simulink model "AirCtl_Mon"  (R2016b)
settings: configuration reference "CodeGenConfigSet" (kept outside this file)
values from neighbouring files (symbols this model uses):
  AirCtl_dnEngTrans_C = Calibration.Parameter    [init_AirCtl_Mon.m]    (also in init_AirCtl_Mon_SIL.m = Simulink.Parameter)
  AirCtl_dqLeadTrans_C = Calibration.Parameter    [init_AirCtl_Mon.m]    (also in init_AirCtl_Mon_SIL.m = Simulink.Parameter)
  AirCtl_drAPPTrans_C = Calibration.Parameter    [init_AirCtl_Mon.m]    (also in init_AirCtl_Mon_SIL.m = Simulink.Parameter)
  AirCtl_facActDesVal_C = Calibration.Parameter    [init_AirCtl_Mon.m]    (also in init_AirCtl_Mon_SIL.m = Simulink.Parameter)
  AirCtl_facEngTempSmkHysCor_CUR = Calibration.Parameter    [init_AirCtl_Mon.m]    (also in init_AirCtl_Mon_SIL.m = Simulink.Parameter)
  AirCtl_facEngTempSmkHysCor_CURX = Calibration.Parameter    [init_AirCtl_Mon.m]    (also in init_AirCtl_Mon_SIL.m = Simulink.Parameter)
  AirCtl_facEnvPresSmkHysCor_CUR = Calibration.Parameter    [init_AirCtl_Mon.m]    (also in init_AirCtl_Mon_SIL.m = Simulink.Parameter)
  AirCtl_facEnvPresSmkHysCor_CURX = Calibration.Parameter    [init_AirCtl_Mon.m]    (also in init_AirCtl_Mon_SIL.m = Simulink.Parameter)
  AirCtl_mMaxDvt_MAP = Calibration.Parameter    [init_AirCtl_Mon.m]    (also in init_AirCtl_Mon_SIL.m = Simulink.Parameter)
  AirCtl_mMaxDvt_MAPX = Calibration.Parameter    [init_AirCtl_Mon.m]    (also in init_AirCtl_Mon_SIL.m = Simulink.Parameter)
  AirCtl_mMaxDvt_MAPY = Calibration.Parameter    [init_AirCtl_Mon.m]    (also in init_AirCtl_Mon_SIL.m = Simulink.Parameter)
  AirCtl_mMinDvt_MAP = Calibration.Parameter    [init_AirCtl_Mon.m]    (also in init_AirCtl_Mon_SIL.m = Simulink.Parameter)
  AirCtl_mMinDvt_MAPX = Calibration.Parameter    [init_AirCtl_Mon.m]    (also in init_AirCtl_Mon_SIL.m = Simulink.Parameter)
  AirCtl_mMinDvt_MAPY = Calibration.Parameter    [init_AirCtl_Mon.m]    (also in init_AirCtl_Mon_SIL.m = Simulink.Parameter)
  AirCtl_nLoIdl_C = Calibration.Parameter    [init_AirCtl_Mon.m]    (also in init_AirCtl_Mon_SIL.m = Simulink.Parameter)
  AirCtl_nOvrRun_C = Calibration.Parameter    [init_AirCtl_Mon.m]    (also in init_AirCtl_Mon_SIL.m = Simulink.Parameter)
  AirCtl_numAirTempMon_C = Calibration.Parameter    [init_AirCtl_Mon.m]    (also in init_AirCtl_Mon_SIL.m = Simulink.Parameter)
  AirCtl_numEngTempMon_C = Calibration.Parameter    [init_AirCtl_Mon.m]    (also in init_AirCtl_Mon_SIL.m = Simulink.Parameter)
  AirCtl_pAirHi_C = Calibration.Parameter    [init_AirCtl_Mon.m]    (also in init_AirCtl_Mon_SIL.m = Simulink.Parameter)
  AirCtl_pAirLo_C = Calibration.Parameter    [init_AirCtl_Mon.m]    (also in init_AirCtl_Mon_SIL.m = Simulink.Parameter)
  AirCtl_qEngTempSmkHysCor_MAP = Calibration.Parameter    [init_AirCtl_Mon.m]    (also in init_AirCtl_Mon_SIL.m = Simulink.Parameter)
  AirCtl_qEngTempSmkHysCor_MAPX = Calibration.Parameter    [init_AirCtl_Mon.m]    (also in init_AirCtl_Mon_SIL.m = Simulink.Parameter)
  AirCtl_qEngTempSmkHysCor_MAPY = Calibration.Parameter    [init_AirCtl_Mon.m]    (also in init_AirCtl_Mon_SIL.m = Simulink.Parameter)
  AirCtl_qEnvPresSmkHysCor_MAP = Calibration.Parameter    [init_AirCtl_Mon.m]    (also in init_AirCtl_Mon_SIL.m = Simulink.Parameter)
  AirCtl_qEnvPresSmkHysCor_MAPX = Calibration.Parameter    [init_AirCtl_Mon.m]    (also in init_AirCtl_Mon_SIL.m = Simulink.Parameter)
  AirCtl_qEnvPresSmkHysCor_MAPY = Calibration.Parameter    [init_AirCtl_Mon.m]    (also in init_AirCtl_Mon_SIL.m = Simulink.Parameter)
  AirCtl_qOvrRun_C = Calibration.Parameter    [init_AirCtl_Mon.m]    (also in init_AirCtl_Mon_SIL.m = Simulink.Parameter)
  AirCtl_qSmkHys_MAP = Calibration.Parameter    [init_AirCtl_Mon.m]    (also in init_AirCtl_Mon_SIL.m = Simulink.Parameter)
  AirCtl_qSmkHys_MAPX = Calibration.Parameter    [init_AirCtl_Mon.m]    (also in init_AirCtl_Mon_SIL.m = Simulink.Parameter)
  AirCtl_qSmkHys_MAPY = Calibration.Parameter    [init_AirCtl_Mon.m]    (also in init_AirCtl_Mon_SIL.m = Simulink.Parameter)
  AirCtl_qSwtSmkHi_C = Calibration.Parameter    [init_AirCtl_Mon.m]    (also in init_AirCtl_Mon_SIL.m = Simulink.Parameter)
  AirCtl_qSwtSmkLo_C = Calibration.Parameter    [init_AirCtl_Mon.m]    (also in init_AirCtl_Mon_SIL.m = Simulink.Parameter)
  AirCtl_rEGRDflVal_CA = Calibration.Parameter    [init_AirCtl_Mon.m]    (also in init_AirCtl_Mon_SIL.m = Simulink.Parameter)
  AirCtl_rTVADflVal_CA = Calibration.Parameter    [init_AirCtl_Mon.m]    (also in init_AirCtl_Mon_SIL.m = Simulink.Parameter)
  AirCtl_stPrioMon_CA = Calibration.Parameter    [init_AirCtl_Mon.m]    (also in init_AirCtl_Mon_SIL.m = Simulink.Parameter)
  AirCtl_swtGovDvtMonEna_C = Calibration.Parameter    [init_AirCtl_Mon.m]    (also in init_AirCtl_Mon_SIL.m = Simulink.Parameter)
  AirCtl_tAirCldHi_C = Calibration.Parameter    [init_AirCtl_Mon.m]    (also in init_AirCtl_Mon_SIL.m = Simulink.Parameter)
  AirCtl_tAirCldLo_C = Calibration.Parameter    [init_AirCtl_Mon.m]    (also in init_AirCtl_Mon_SIL.m = Simulink.Parameter)
  AirCtl_tAirWrmHi_C = Calibration.Parameter    [init_AirCtl_Mon.m]    (also in init_AirCtl_Mon_SIL.m = Simulink.Parameter)
  AirCtl_tAirWrmLo_C = Calibration.Parameter    [init_AirCtl_Mon.m]    (also in init_AirCtl_Mon_SIL.m = Simulink.Parameter)
  AirCtl_tClntCldHi_C = Calibration.Parameter    [init_AirCtl_Mon.m]    (also in init_AirCtl_Mon_SIL.m = Simulink.Parameter)
  AirCtl_tClntCldLo_C = Calibration.Parameter    [init_AirCtl_Mon.m]    (also in init_AirCtl_Mon_SIL.m = Simulink.Parameter)
  AirCtl_tClntWrmHi_C = Calibration.Parameter    [init_AirCtl_Mon.m]    (also in init_AirCtl_Mon_SIL.m = Simulink.Parameter)
  AirCtl_tClntWrmLo_C = Calibration.Parameter    [init_AirCtl_Mon.m]    (also in init_AirCtl_Mon_SIL.m = Simulink.Parameter)
  AirCtl_tiCldStrt_CUR = Calibration.Parameter    [init_AirCtl_Mon.m]    (also in init_AirCtl_Mon_SIL.m = Simulink.Parameter)
  AirCtl_tiCldStrt_CURX = Calibration.Parameter    [init_AirCtl_Mon.m]    (also in init_AirCtl_Mon_SIL.m = Simulink.Parameter)
  AirCtl_tiClth_C = Calibration.Parameter    [init_AirCtl_Mon.m]    (also in init_AirCtl_Mon_SIL.m = Simulink.Parameter)
  AirCtl_tiDynSmkDly_C = Calibration.Parameter    [init_AirCtl_Mon.m]    (also in init_AirCtl_Mon_SIL.m = Simulink.Parameter)
  AirCtl_tiGovDvtMaxDebDef_C = Calibration.Parameter    [init_AirCtl_Mon.m]    (also in init_AirCtl_Mon_SIL.m = Simulink.Parameter)
  AirCtl_tiGovDvtMaxDebOk_C = Calibration.Parameter    [init_AirCtl_Mon.m]    (also in init_AirCtl_Mon_SIL.m = Simulink.Parameter)
  AirCtl_tiGovDvtMinDebDef_C = Calibration.Parameter    [init_AirCtl_Mon.m]    (also in init_AirCtl_Mon_SIL.m = Simulink.Parameter)
  AirCtl_tiGovDvtMinDebOk_C = Calibration.Parameter    [init_AirCtl_Mon.m]    (also in init_AirCtl_Mon_SIL.m = Simulink.Parameter)
  AirCtl_tiLoIdl_C = Calibration.Parameter    [init_AirCtl_Mon.m]    (also in init_AirCtl_Mon_SIL.m = Simulink.Parameter)
  AirCtl_tiStatSmkDly_C = Calibration.Parameter    [init_AirCtl_Mon.m]    (also in init_AirCtl_Mon_SIL.m = Simulink.Parameter)
  AirCtl_tiTransDly_C = Calibration.Parameter    [init_AirCtl_Mon.m]    (also in init_AirCtl_Mon_SIL.m = Simulink.Parameter)
  AirCtl_uBattThres_C = Calibration.Parameter    [init_AirCtl_Mon.m]    (also in init_AirCtl_Mon_SIL.m = Simulink.Parameter)
  ASMod_numBnk_C = Calibration.Parameter    [init_AirCtl_Mon.m]    (also in init_AirCtl_Mon_SIL.m = Simulink.Parameter)
  Epm_numCyl_C = Calibration.Parameter    [init_AirCtl_Mon.m]    (also in init_AirCtl_Mon_SIL.m = Simulink.Parameter)
undefined symbols (not defined in the file or in its folder): AirCtl_Mon_DT, EngState_conv, Switch_conv
libraries: simulink x45, CXLib x23
(part 3 of 4)

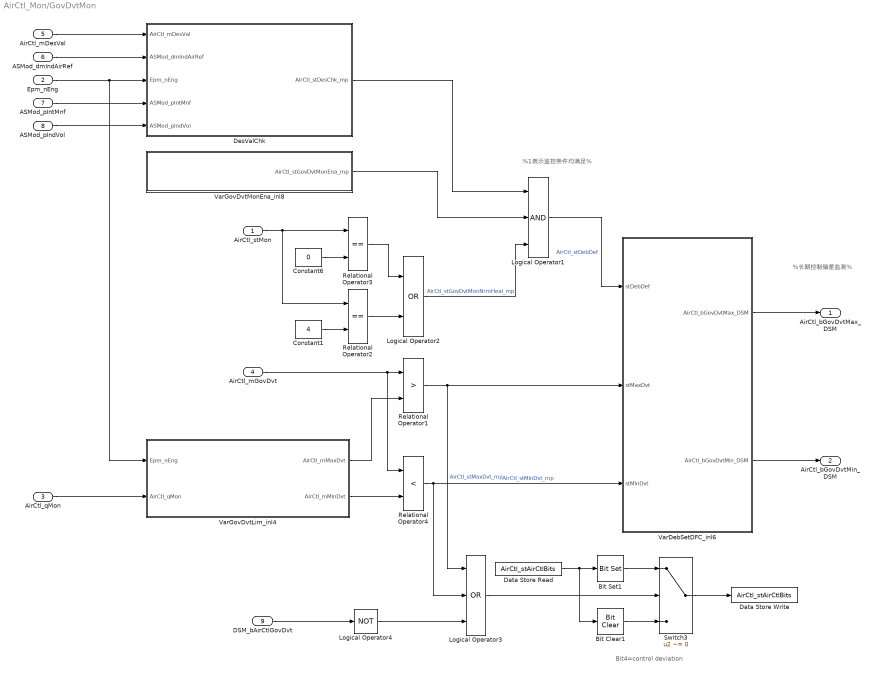
== system AirCtl_Mon/GovDvtMon ==
  note: %长期控制偏差监测%
  note: %1表示监控条件均满足%
  note: Bit4=control deviation
  AirCtl_stMon : Inport
  Epm_nEng : Inport  Port=2
  AirCtl_qMon : Inport  Port=3
  AirCtl_mGovDvt : Inport  Port=4
  AirCtl_mDesVal : Inport  Port=5
  ASMod_dmIndAirRef : Inport  Port=6
  ASMod_pIntMnf : Inport  Port=7
  ASMod_pIndVol : Inport  Port=8
  DSM_bAirCtlGovDvt : Inport  Description=Status of Fid_AirCtlGovDvt  Port=9  OutMin=0  OutMax=1
  Bit Clear1 : simulink/Logic and Bit Operations/Bit Clear  iBit=4
  Bit Set1 : simulink/Logic and Bit Operations/Bit Set  iBit=4
  Constant1 : Constant  Value=4  OutDataTypeStr=Inherit: Inherit via back propagation
  Constant6 : Constant  Value=0  OutDataTypeStr=Inherit: Inherit via back propagation
  Data Store Read : DataStoreRead  DataStoreName=AirCtl_stAirCtlBits
  Data Store Write : DataStoreWrite  DataStoreName=AirCtl_stAirCtlBits
  DesValChk : Subsystem
  Logical Operator1 : Logic  Inputs=3  OutDataTypeStr=boolean
  Logical Operator2 : Logic  Operator=OR  OutDataTypeStr=boolean
  Logical Operator3 : Logic  Operator=OR  Inputs=3  OutDataTypeStr=boolean
  Logical Operator4 : Logic  Operator=NOT  AllPortsSameDT=off  OutDataTypeStr=boolean
  Relational Operator1 : RelationalOperator  Operator=>  OutDataTypeStr=boolean  RndMeth=Simplest  InputSameDT=on
  Relational Operator2 : RelationalOperator  Operator===  OutDataTypeStr=boolean  RndMeth=Simplest  InputSameDT=on
  Relational Operator3 : RelationalOperator  Operator===  OutDataTypeStr=boolean  RndMeth=Simplest  InputSameDT=on
  Relational Operator4 : RelationalOperator  Operator=<  OutDataTypeStr=boolean  RndMeth=Simplest  InputSameDT=on
  Switch3 : Switch  Criteria=u2 ~= 0  SaturateOnIntegerOverflow=on  InputSameDT=on
  VarDebSetDFC_inl6 : Subsystem
  VarGovDvtLim_inl4 : Subsystem
  VarGovDvtMonEna_inl8 : Subsystem
  AirCtl_bGovDvtMax_DSM : Outport  Description=DFC of AirCtl_bGovDvtMax  OutMin=0  OutMax=1
  AirCtl_bGovDvtMin_DSM : Outport  Description=DFC of AirCtl_bGovDvtMin  Port=2  OutMin=0  OutMax=1
  wires:
  Logical Operator4/1 -> Logical Operator3/3
  Switch3/1 -> Data Store Write/1
  DSM_bAirCtlGovDvt/1 -> Logical Operator4/1
  AirCtl_mGovDvt/1 -> Relational Operator1/1, Relational Operator4/1
  Data Store Read/1 -> Bit Set1/1, Bit Clear1/1
  Bit Clear1/1 -> Switch3/3
  Logical Operator3/1 -> Switch3/2
  Bit Set1/1 -> Switch3/1
  ASMod_pIndVol/1 -> DesValChk/5(ASMod_pIndVol)
  Logical Operator1/1 -> VarDebSetDFC_inl6/1(stDebDef)  "AirCtl_stDebDef"
  ASMod_pIntMnf/1 -> DesValChk/4(ASMod_pIntMnf)
  Epm_nEng/1 -> DesValChk/3(Epm_nEng), VarGovDvtLim_inl4/1(Epm_nEng)
  Constant6/1 -> Relational Operator3/2
  DesValChk/1(AirCtl_stDesChk_mp) -> Logical Operator1/1
  ASMod_dmIndAirRef/1 -> DesValChk/2(ASMod_dmIndAirRef)
  VarGovDvtMonEna_inl8/1(AirCtl_stGovDvtMonEna_mp) -> Logical Operator1/2
  Relational Operator4/1 -> VarDebSetDFC_inl6/3(stMinDvt), Logical Operator3/2  "AirCtl_stMinDvt_mp"
  AirCtl_mDesVal/1 -> DesValChk/1(AirCtl_mDesVal)
  Relational Operator3/1 -> Logical Operator2/1
  VarGovDvtLim_inl4/1(AirCtl_mMaxDvt) -> Relational Operator1/2
  VarGovDvtLim_inl4/2(AirCtl_mMinDvt) -> Relational Operator4/2
  AirCtl_stMon/1 -> Relational Operator2/1, Relational Operator3/1
  Relational Operator1/1 -> VarDebSetDFC_inl6/2(stMaxDvt), Logical Operator3/1  "AirCtl_stMaxDvt_mp"
  AirCtl_qMon/1 -> VarGovDvtLim_inl4/2(AirCtl_qMon)
  VarDebSetDFC_inl6/1(AirCtl_bGovDvtMax_DSM) -> AirCtl_bGovDvtMax_DSM/1
  VarDebSetDFC_inl6/2(AirCtl_bGovDvtMin_DSM) -> AirCtl_bGovDvtMin_DSM/1
  Constant1/1 -> Relational Operator2/2
  Relational Operator2/1 -> Logical Operator2/2
  Logical Operator2/1 -> Logical Operator1/3  "AirCtl_stGovDvtMonNrmHeal_mp"

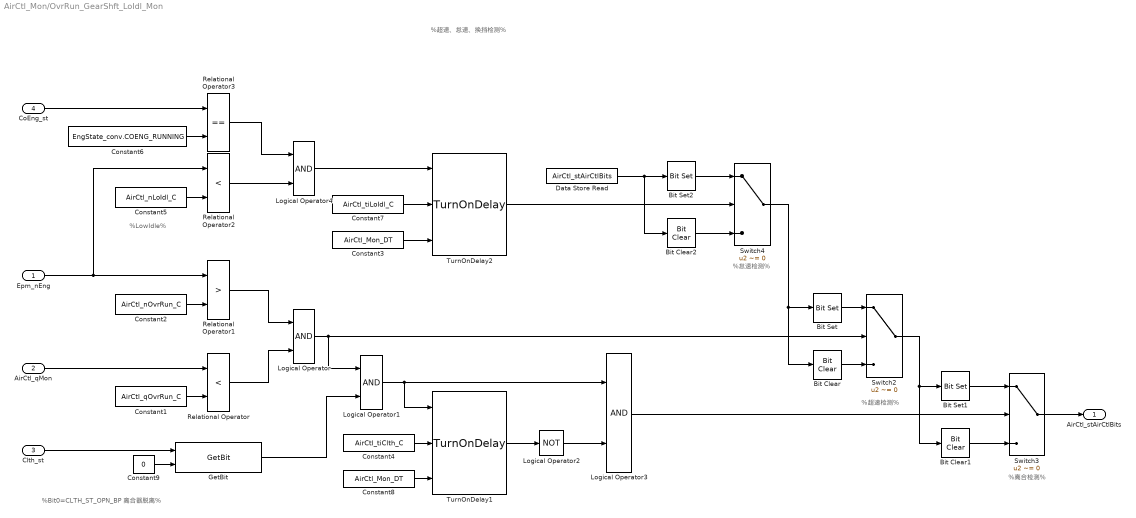
== system AirCtl_Mon/OvrRun_GearShft_LoIdl_Mon ==
  note: %超速、怠速、换挡检测%
  note: %Bit0=CLTH_ST_OPN_BP 离合器脱离%
  note: %LowIdle%
  note: %怠速检测%
  note: %超速检测%
  note: %离合检测%
  Epm_nEng : Inport
  AirCtl_qMon : Inport  Port=2
  Clth_st : Inport  Port=3
  CoEng_st : Inport  Port=4
  Bit Clear : simulink/Logic and Bit Operations/Bit Clear  iBit=1
  Bit Clear1 : simulink/Logic and Bit Operations/Bit Clear  iBit=2
  Bit Clear2 : simulink/Logic and Bit Operations/Bit Clear  iBit=3
  Bit Set : simulink/Logic and Bit Operations/Bit Set  iBit=1
  Bit Set1 : simulink/Logic and Bit Operations/Bit Set  iBit=2
  Bit Set2 : simulink/Logic and Bit Operations/Bit Set  iBit=3
  Constant1 : Constant  Value=AirCtl_qOvrRun_C
  Constant2 : Constant  Value=AirCtl_nOvrRun_C
  Constant3 : Constant  Value=AirCtl_Mon_DT
  Constant4 : Constant  Value=AirCtl_tiClth_C
  Constant5 : Constant  Value=AirCtl_nLoIdl_C
  Constant6 : Constant  Value=EngState_conv.COENG_RUNNING  OutDataTypeStr=Inherit: Inherit via back propagation
  Constant7 : Constant  Value=AirCtl_tiLoIdl_C
  Constant8 : Constant  Value=AirCtl_Mon_DT
  Constant9 : Constant  Value=0  OutDataTypeStr=uint8
  Data Store Read : DataStoreRead  DataStoreName=AirCtl_stAirCtlBits
  GetBit : CXLib/GetBit  dataTypeString=uint8  dataLength=0
      settings: AttributesFormatString=Get bit from %<dataTypeString>
  Logical Operator{,1,3..4} (4 alike) : Logic  OutDataTypeStr=boolean
  Logical Operator2 : Logic  Operator=NOT  AllPortsSameDT=off  OutDataTypeStr=boolean
  Relational Operator : RelationalOperator  Operator=<  OutDataTypeStr=boolean  RndMeth=Simplest  InputSameDT=on
  Relational Operator1 : RelationalOperator  Operator=>  OutDataTypeStr=boolean  RndMeth=Simplest  InputSameDT=on
  Relational Operator2 : RelationalOperator  Operator=<  OutDataTypeStr=boolean  RndMeth=Simplest  InputSameDT=on
  Relational Operator3 : RelationalOperator  Operator===  OutDataTypeStr=boolean  RndMeth=Simplest  InputSameDT=on
  Switch2 : Switch  Criteria=u2 ~= 0  SaturateOnIntegerOverflow=on  InputSameDT=on
  Switch3 : Switch  Criteria=u2 ~= 0  SaturateOnIntegerOverflow=on  InputSameDT=on
  Switch4 : Switch  Criteria=u2 ~= 0  SaturateOnIntegerOverflow=on  InputSameDT=on
  TurnOnDelay1 : CXLib/TurnOnDelay
  TurnOnDelay2 : CXLib/TurnOnDelay
  AirCtl_stAirCtlBits : Outport
  wires:
  Switch3/1 -> AirCtl_stAirCtlBits/1
  Constant3/1 -> TurnOnDelay2/3
  Constant8/1 -> TurnOnDelay1/3
  GetBit/1 -> Logical Operator1/2
  Data Store Read/1 -> Bit Set2/1, Bit Clear2/1
  Switch2/1 -> Bit Clear1/1, Bit Set1/1
  Bit Clear2/1 -> Switch4/3
  Bit Set2/1 -> Switch4/1
  Bit Clear1/1 -> Switch3/3
  Bit Set1/1 -> Switch3/1
  TurnOnDelay2/1 -> Switch4/2
  Logical Operator3/1 -> Switch3/2
  Bit Clear/1 -> Switch2/3
  Bit Set/1 -> Switch2/1
  Switch4/1 -> Bit Set/1, Bit Clear/1
  Logical Operator4/1 -> TurnOnDelay2/1
  Constant7/1 -> TurnOnDelay2/2
  CoEng_st/1 -> Relational Operator3/1
  Constant6/1 -> Relational Operator3/2
  Relational Operator3/1 -> Logical Operator4/1
  Relational Operator2/1 -> Logical Operator4/2
  Constant5/1 -> Relational Operator2/2
  Logical Operator2/1 -> Logical Operator3/2
  TurnOnDelay1/1 -> Logical Operator2/1
  Constant4/1 -> TurnOnDelay1/2
  Logical Operator1/1 -> TurnOnDelay1/1, Logical Operator3/1
  Clth_st/1 -> GetBit/1
  Logical Operator/1 -> Switch2/2, Logical Operator1/1
  Relational Operator/1 -> Logical Operator/2
  Relational Operator1/1 -> Logical Operator/1
  Epm_nEng/1 -> Relational Operator2/1, Relational Operator1/1
  Constant2/1 -> Relational Operator1/2
  Constant1/1 -> Relational Operator/2
  AirCtl_qMon/1 -> Relational Operator/1
  Constant9/1 -> GetBit/2

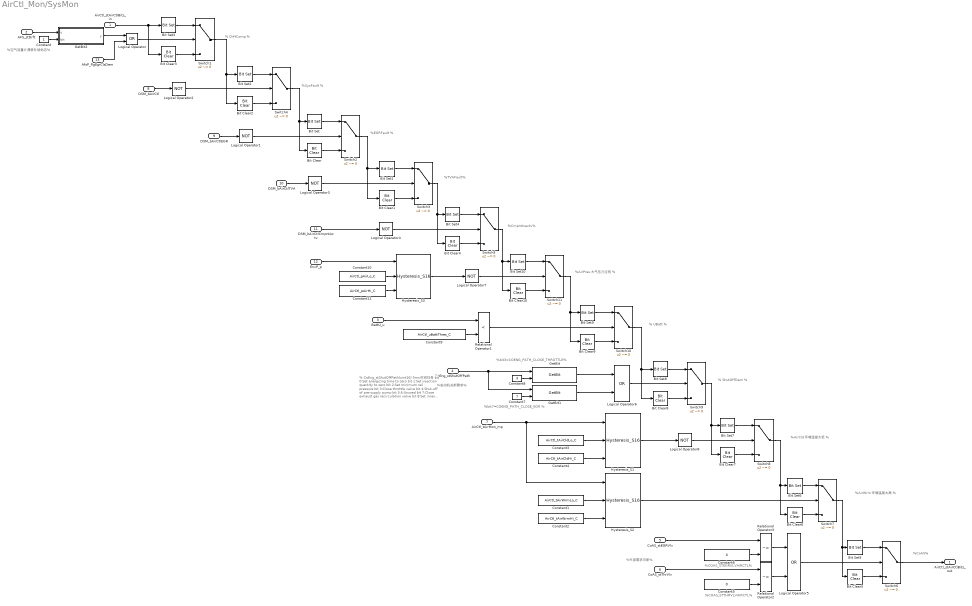
== system AirCtl_Mon/SysMon ==
  note: % CoEng_stShutOffPath(uint16) 5ms时间任务
      | bit 0:Set energizing time to zero
      | bit 1:Set injection quantity to zero
      | bit 2:Set minimum rail pressure
      | bit 3:Close throttle valve
      | bit 4:Shut-off of pre-supply pump
      | bit 5,6:Unused
      | bit 7:Close exhaust gas recirculation valve
      | bit 8:Set inner torque to zero %
  note: %bit7=COENG_PATH_CLOSE_EGR %
  note: % DrftComp %
  note: %AirPres 大气压力过低 %
  note: % UBatt %
  note: % ShutOffDem %
  note: %AirCld 环境温度太低 %
  note: %AirWrm 环境温度太高 %
  note: %CoAS%
  note: %CmpntInactv%
  note: %SysFault %
  note: %EGRFault %
  note: %TVAFault%
  note: %空气流量计漂移补偿标志%
  note: %外部需求中断%
  note: %发动机关断需求%
  note: %bit3=COENG_PATH_CLOSE_THROTTLE%
  note: %COAS_STEGRVLVAIRCTL%
  note: %COAS_STTHRVLVAIRCTL%
  AirCtl_stAirCtlBits_in : Inport
  AFS_stDrft : Inport  Port=2
  BattU_u : Inport  Port=3
  CoEng_stShutOffPath : Inport  Port=4
  CoAS_stEGRVlv : Inport  Port=5
  CoAS_stThrVlv : Inport  Port=6
  " AirCtl_tAirMon_mp" : Inport  Port=7
  DSM_bAirCtl : Inport  Description=Status of Fid_AirCtl  Port=8  OutMin=0  OutMax=1
  DSM_bAirCtlEGR : Inport  Description=Status of Fid_AirCtlEGR  Port=9  OutMin=0  OutMax=1
  DSM_bAirCtlTVA : Inport  Description=Status of Fid_AirCtlTVA  Port=10  OutMin=0  OutMax=1
  DSM_bAirCtlCmpntActv : Inport  Description=Status of Fid_AirCtlCmpntActv  Port=11  OutMin=0  OutMax=1
  EnvP_p : Inport  Port=12
  AfsP_flgEgrClsDem : Inport  Port=13
  Bit Clear : simulink/Logic and Bit Operations/Bit Clear  iBit=7
  Bit Clear1 : simulink/Logic and Bit Operations/Bit Clear  iBit=8
  Bit Clear10 : simulink/Logic and Bit Operations/Bit Clear  iBit=10
  Bit Clear2 : simulink/Logic and Bit Operations/Bit Clear  iBit=6
  Bit Clear3 : simulink/Logic and Bit Operations/Bit Clear  iBit=5
  Bit Clear4 : simulink/Logic and Bit Operations/Bit Clear  iBit=9
  Bit Clear5 : simulink/Logic and Bit Operations/Bit Clear  iBit=21
  Bit Clear6 : simulink/Logic and Bit Operations/Bit Clear  iBit=14
  Bit Clear7 : simulink/Logic and Bit Operations/Bit Clear  iBit=13
  Bit Clear8 : simulink/Logic and Bit Operations/Bit Clear  iBit=12
  Bit Clear9 : simulink/Logic and Bit Operations/Bit Clear  iBit=11
  Bit Set : simulink/Logic and Bit Operations/Bit Set  iBit=7
  Bit Set1 : simulink/Logic and Bit Operations/Bit Set  iBit=8
  Bit Set10 : simulink/Logic and Bit Operations/Bit Set  iBit=10
  Bit Set2 : simulink/Logic and Bit Operations/Bit Set  iBit=6
  Bit Set3 : simulink/Logic and Bit Operations/Bit Set  iBit=5
  Bit Set4 : simulink/Logic and Bit Operations/Bit Set  iBit=9
  Bit Set5 : simulink/Logic and Bit Operations/Bit Set  iBit=21
  Bit Set6 : simulink/Logic and Bit Operations/Bit Set  iBit=14
  Bit Set7 : simulink/Logic and Bit Operations/Bit Set  iBit=13
  Bit Set8 : simulink/Logic and Bit Operations/Bit Set  iBit=12
  Bit Set9 : simulink/Logic and Bit Operations/Bit Set  iBit=11
  Constant : Constant  OutDataTypeStr=uint8
  Constant1 : Constant  Value=AirCtl_tAirWrmLo_C
  Constant10 : Constant  Value=AirCtl_pAirLo_C
  Constant11 : Constant  Value=AirCtl_pAirHi_C
  Constant2 : Constant  Value=AirCtl_tAirWrmHi_C
  Constant3 : Constant  Value=AirCtl_tAirCldLo_C
  Constant4 : Constant  Value=AirCtl_tAirCldHi_C
  Constant5 : Constant  Value=0  OutDataTypeStr=Inherit: Inherit via back propagation
  Constant6 : Constant  Value=0  OutDataTypeStr=Inherit: Inherit via back propagation
  Constant7 : Constant  Value=7  OutDataTypeStr=uint8
  Constant8 : Constant  Value=3  OutDataTypeStr=uint8
  Constant9 : Constant  Value=AirCtl_uBattThres_C
  GetBit : CXLib/GetBit  dataTypeString=uint16  dataLength=0
      settings: AttributesFormatString=Get bit from %<dataTypeString>
  GetBit1 : CXLib/GetBit  dataTypeString=uint16  dataLength=0
      settings: AttributesFormatString=Get bit from %<dataTypeString>
  GetBit2 : Subsystem  mask(GetBit){dataTypeString=uint8, dataLength=0}
      mask prompts: dataTypeString "Input Data Type"; dataLength "DataType Length"
      mask help:
      | Acquires the value of the bit specified by the position (zero indexed).
      |
      | Output is always boolean.
      |
      | INPUTS:
      | u - input value
      | bit - position of bit to get (uint8)
      |
      | OUTPUTS:
      | y - output value
      mask init: same as AirCtl_Mon/CheckPrio/GetBit1
      settings: AttributesFormatString=Get bit from %<dataTypeString>
      mask Display: image(imread('GETBIT.jpg'),[0.2,0.2,0.6,0.6]);
  Hysteresis_S1 : CXLib/Hysteresis_S16
  Hysteresis_S2 : CXLib/Hysteresis_S16
  Hysteresis_S3 : CXLib/Hysteresis_S16
  Logical Operator : Logic  Operator=OR  AllPortsSameDT=off  OutDataTypeStr=boolean
  Logical Operator{1..4,7..8} (6 alike) : Logic  Operator=NOT  AllPortsSameDT=off  OutDataTypeStr=boolean
  Logical Operator5 : Logic  Operator=OR  OutDataTypeStr=boolean
  Logical Operator6 : Logic  Operator=OR  OutDataTypeStr=boolean
  Relational Operator1 : RelationalOperator  Operator=<  OutDataTypeStr=boolean  RndMeth=Simplest  InputSameDT=on
  Relational Operator2 : RelationalOperator  Operator=~=  OutDataTypeStr=boolean  RndMeth=Simplest  InputSameDT=on
  Relational Operator3 : RelationalOperator  Operator=~=  OutDataTypeStr=boolean  RndMeth=Simplest  InputSameDT=on
  Switch{1..11} (11 alike) : Switch  Criteria=u2 ~= 0  SaturateOnIntegerOverflow=on  InputSameDT=on
  AirCtl_stAirCtlBits_out : Outport
  wires:
  " AirCtl_tAirMon_mp"/1 -> Hysteresis_S2/1, Hysteresis_S1/1
  Switch11/1 -> Bit Clear9/1, Bit Set9/1
  DSM_bAirCtlCmpntActv/1 -> Logical Operator4/1
  DSM_bAirCtlTVA/1 -> Logical Operator3/1
  DSM_bAirCtl/1 -> Logical Operator2/1
  Bit Clear3/1 -> Switch1/3
  Switch1/1 -> Bit Set2/1, Bit Clear2/1
  Switch4/1 -> Bit Clear/1, Bit Set/1
  Switch2/1 -> Bit Clear1/1, Bit Set1/1
  Switch3/1 -> Bit Clear4/1, Bit Set4/1
  Switch6/1 -> AirCtl_stAirCtlBits_out/1
  Switch7/1 -> Bit Clear5/1, Bit Set5/1
  Switch8/1 -> Bit Clear6/1, Bit Set6/1
  Switch9/1 -> Bit Clear7/1, Bit Set7/1
  Switch10/1 -> Bit Clear8/1, Bit Set8/1
  AirCtl_stAirCtlBits_in/1 -> Bit Clear3/1, Bit Set3/1
  Logical Operator8/1 -> Switch8/2
  Logical Operator7/1 -> Switch11/2
  Hysteresis_S3/1 -> Logical Operator7/1
  Bit Clear10/1 -> Switch11/3
  Bit Set10/1 -> Switch11/1
  Constant11/1 -> Hysteresis_S3/3
  Constant10/1 -> Hysteresis_S3/2
  EnvP_p/1 -> Hysteresis_S3/1
  Relational Operator1/1 -> Switch10/2
  Bit Clear9/1 -> Switch10/3
  Bit Set9/1 -> Switch10/1
  Constant9/1 -> Relational Operator1/2
  BattU_u/1 -> Relational Operator1/1
  Logical Operator6/1 -> Switch9/2
  Bit Clear8/1 -> Switch9/3
  Bit Set8/1 -> Switch9/1
  CoEng_stShutOffPath/1 -> GetBit1/1, GetBit/1
  Hysteresis_S1/1 -> Logical Operator8/1
  Bit Clear7/1 -> Switch8/3
  Bit Set7/1 -> Switch8/1
  Constant4/1 -> Hysteresis_S1/3
  Constant3/1 -> Hysteresis_S1/2
  Hysteresis_S2/1 -> Switch7/2
  Bit Clear6/1 -> Switch7/3
  Bit Set6/1 -> Switch7/1
  Bit Clear5/1 -> Switch6/3
  Bit Set5/1 -> Switch6/1
  Constant2/1 -> Hysteresis_S2/3
  Constant1/1 -> Hysteresis_S2/2
  CoAS_stEGRVlv/1 -> Relational Operator3/1
  Logical Operator5/1 -> Switch6/2
  Constant6/1 -> Relational Operator3/2
  Relational Operator3/1 -> Logical Operator5/1
  Relational Operator2/1 -> Logical Operator5/2
  Constant5/1 -> Relational Operator2/2
  CoAS_stThrVlv/1 -> Relational Operator2/1
  Logical Operator4/1 -> Switch5/2
  Switch5/1 -> Bit Clear10/1, Bit Set10/1
  Bit Clear4/1 -> Switch5/3
  Bit Set4/1 -> Switch5/1
  Logical Operator3/1 -> Switch3/2
  Logical Operator1/1 -> Switch2/2
  Bit Set3/1 -> Switch1/1
  Logical Operator2/1 -> Switch4/2
  DSM_bAirCtlEGR/1 -> Logical Operator1/1
  Bit Clear2/1 -> Switch4/3
  Bit Set2/1 -> Switch4/1
  Bit Clear1/1 -> Switch3/3
  Bit Set1/1 -> Switch3/1
  Bit Clear/1 -> Switch2/3
  Bit Set/1 -> Switch2/1
  AFS_stDrft/1 -> GetBit2/1(u)
  Constant/1 -> GetBit2/2(bit)
  Constant7/1 -> GetBit1/2
  Constant8/1 -> GetBit/2
  Logical Operator/1 -> Switch1/2
  AfsP_flgEgrClsDem/1 -> Logical Operator/2
  GetBit/1 -> Logical Operator6/1
  GetBit1/1 -> Logical Operator6/2
  GetBit2/1(y) -> Logical Operator/1

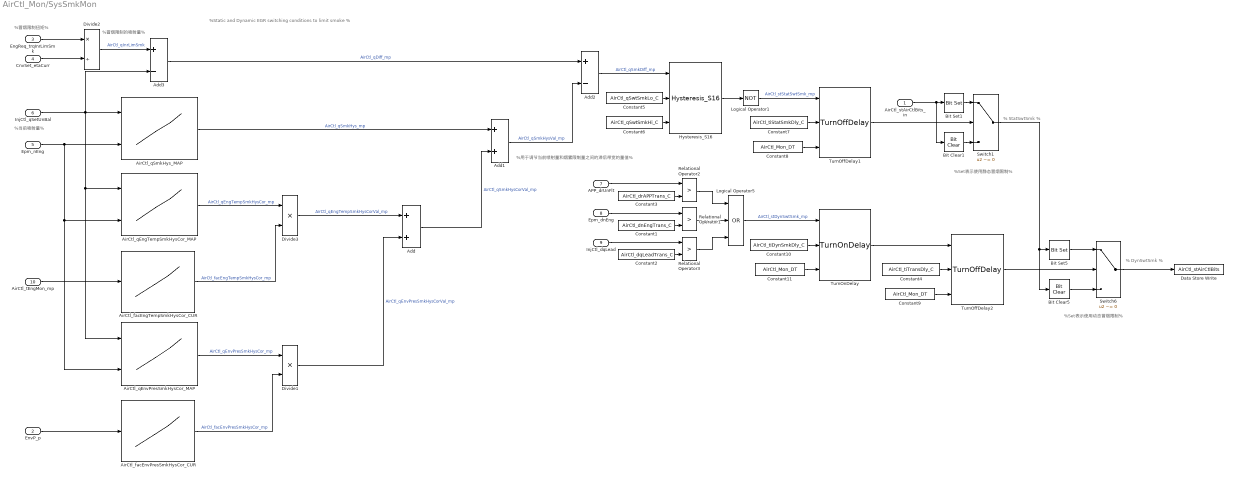
== system AirCtl_Mon/SysSmkMon ==
  note: %Set表示使用动态冒烟限制%
  note: % StatSwtSmk %
  note: % DynSwtSmk %
  note: %Static and Dynamic EGR switching conditions to limit smoke %
  note: %冒烟限制扭矩%
  note: %Set表示使用静态冒烟限制%
  note: %冒烟限制的喷射量%
  note: %当前喷射量%
  note: %用于调节当前喷射量和烟雾限制量之间的滞后带宽的量值%
  AirCtl_stAirCtlBits_in : Inport
  EnvP_p : Inport  Port=2
  EngReq_trqInrLimSmk : Inport  Port=3
  CnvSet_etaCurr : Inport  Port=4
  Epm_nEng : Inport  Port=5
  InjCtl_qSetUnBal : Inport  Port=6
  APP_drUnFlt : Inport  Port=7
  Epm_dnEng : Inport  Port=8
  InjCtl_dqLead : Inport  Port=9
  AirCtl_tEngMon_mp : Inport  Port=10
  Add : Sum  SaturateOnIntegerOverflow=on  InputSameDT=on
  Add1 : Sum  SaturateOnIntegerOverflow=on  InputSameDT=on
  Add2 : Sum  Inputs=+-  SaturateOnIntegerOverflow=on  InputSameDT=on
  Add3 : Sum  Inputs=+-  SaturateOnIntegerOverflow=on  InputSameDT=on
  AirCtl_facEngTempSmkHysCor_CUR : Lookup_n-D  NumberOfTableDimensions=1  BreakpointsForDimension1=AirCtl_facEngTempSmkHysCor_CURX  BeginIndexSearchUsingPreviousIndexResult=on  Table=AirCtl_facEngTempSmkHysCor_CUR  TableDataTypeStr=Inherit: Inherit from 'Table data'  ExtrapMethod=Clip  UseLastTableValue=on  InternalRulePriority=Speed  OutDataTypeStr=Inherit: Inherit from 'Table data'  RndMeth=Simplest  SaturateOnIntegerOverflow=on
  AirCtl_facEnvPresSmkHysCor_CUR : Lookup_n-D  NumberOfTableDimensions=1  BreakpointsForDimension1=AirCtl_facEnvPresSmkHysCor_CURX  BeginIndexSearchUsingPreviousIndexResult=on  Table=AirCtl_facEnvPresSmkHysCor_CUR  TableDataTypeStr=Inherit: Inherit from 'Table data'  ExtrapMethod=Clip  UseLastTableValue=on  InternalRulePriority=Speed  OutDataTypeStr=Inherit: Inherit from 'Table data'  RndMeth=Simplest  SaturateOnIntegerOverflow=on
  AirCtl_qEngTempSmkHysCor_MAP : Lookup_n-D  BreakpointsForDimension1=AirCtl_qEngTempSmkHysCor_MAPY  BreakpointsForDimension2=AirCtl_qEngTempSmkHysCor_MAPX  BeginIndexSearchUsingPreviousIndexResult=on  Table=AirCtl_qEngTempSmkHysCor_MAP  TableDataTypeStr=Inherit: Inherit from 'Table data'  ExtrapMethod=Clip  UseLastTableValue=on  InternalRulePriority=Speed  OutDataTypeStr=Inherit: Inherit from 'Table data'  RndMeth=Simplest  SaturateOnIntegerOverflow=on
  AirCtl_qEnvPresSmkHysCor_MAP : Lookup_n-D  BreakpointsForDimension1=AirCtl_qEnvPresSmkHysCor_MAPY  BreakpointsForDimension2=AirCtl_qEnvPresSmkHysCor_MAPX  BeginIndexSearchUsingPreviousIndexResult=on  Table=AirCtl_qEnvPresSmkHysCor_MAP  TableDataTypeStr=Inherit: Inherit from 'Table data'  ExtrapMethod=Clip  UseLastTableValue=on  InternalRulePriority=Speed  OutDataTypeStr=Inherit: Inherit from 'Table data'  RndMeth=Simplest  SaturateOnIntegerOverflow=on
  AirCtl_qSmkHys_MAP : Lookup_n-D  BreakpointsForDimension1=AirCtl_qSmkHys_MAPY  BreakpointsForDimension2=AirCtl_qSmkHys_MAPX  BeginIndexSearchUsingPreviousIndexResult=on  Table=AirCtl_qSmkHys_MAP  TableDataTypeStr=Inherit: Inherit from 'Table data'  ExtrapMethod=Clip  UseLastTableValue=on  InternalRulePriority=Speed  OutDataTypeStr=Inherit: Inherit from 'Table data'  RndMeth=Simplest  SaturateOnIntegerOverflow=on
  Bit Clear1 : simulink/Logic and Bit Operations/Bit Clear  iBit=28
  Bit Clear5 : simulink/Logic and Bit Operations/Bit Clear  iBit=29
  Bit Set1 : simulink/Logic and Bit Operations/Bit Set  iBit=28
  Bit Set5 : simulink/Logic and Bit Operations/Bit Set  iBit=29
  Constant1 : Constant  Value=AirCtl_dnEngTrans_C
  Constant10 : Constant  Value=AirCtl_tiDynSmkDly_C
  Constant11 : Constant  Value=AirCtl_Mon_DT
  Constant2 : Constant  Value=AirCtl_dqLeadTrans_C
  Constant3 : Constant  Value=AirCtl_drAPPTrans_C
  Constant4 : Constant  Value=AirCtl_tiTransDly_C
  Constant5 : Constant  Value=AirCtl_qSwtSmkLo_C
  Constant6 : Constant  Value=AirCtl_qSwtSmkHi_C
  Constant7 : Constant  Value=AirCtl_tiStatSmkDly_C
  Constant8 : Constant  Value=AirCtl_Mon_DT
  Constant9 : Constant  Value=AirCtl_Mon_DT
  Data Store Write : DataStoreWrite  DataStoreName=AirCtl_stAirCtlBits
  Divide1 : Product  Inputs=**  OutDataTypeStr=Inherit: Inherit via back propagation  SaturateOnIntegerOverflow=on
  Divide2 : Product  Inputs=*/  OutDataTypeStr=Inherit: Inherit via back propagation  SaturateOnIntegerOverflow=on
  Divide3 : Product  Inputs=**  OutDataTypeStr=Inherit: Inherit via back propagation  SaturateOnIntegerOverflow=on
  Hysteresis_S16 : CXLib/Hysteresis_S16
  Logical Operator1 : Logic  Operator=NOT  Inputs=3  AllPortsSameDT=off  OutDataTypeStr=boolean
  Logical Operator5 : Logic  Operator=OR  Inputs=3  OutDataTypeStr=boolean
  Relational Operator1 : RelationalOperator  Operator=>  OutDataTypeStr=boolean  RndMeth=Simplest  InputSameDT=on
  Relational Operator2 : RelationalOperator  Operator=>  OutDataTypeStr=boolean  RndMeth=Simplest  InputSameDT=on
  Relational Operator3 : RelationalOperator  Operator=>  OutDataTypeStr=boolean  RndMeth=Simplest  InputSameDT=on
  Switch1 : Switch  Criteria=u2 ~= 0  SaturateOnIntegerOverflow=on  InputSameDT=on
  Switch6 : Switch  Criteria=u2 ~= 0  SaturateOnIntegerOverflow=on  InputSameDT=on
  TurnOffDelay1 : CXLib/TurnOffDelay
  TurnOffDelay2 : CXLib/TurnOffDelay
  TurnOnDelay : CXLib/TurnOnDelay
  wires:
  CnvSet_etaCurr/1 -> Divide2/2
  EngReq_trqInrLimSmk/1 -> Divide2/1
  Switch6/1 -> Data Store Write/1
  Constant8/1 -> TurnOffDelay1/3
  Constant9/1 -> TurnOffDelay2/3
  Switch1/1 -> Bit Set5/1, Bit Clear5/1
  AirCtl_stAirCtlBits_in/1 -> Bit Set1/1, Bit Clear1/1
  Bit Clear1/1 -> Switch1/3
  Bit Set1/1 -> Switch1/1
  TurnOffDelay1/1 -> Switch1/2
  Constant7/1 -> TurnOffDelay1/2
  Logical Operator1/1 -> TurnOffDelay1/1  "AirCtl_stStatSwtSmk_mp"
  Hysteresis_S16/1 -> Logical Operator1/1
  Constant6/1 -> Hysteresis_S16/3
  Constant5/1 -> Hysteresis_S16/2
  Add2/1 -> Hysteresis_S16/1  "AirCtl_qSmkDiff_mp"
  Add3/1 -> Add2/1  "AirCtl_qDiff_mp"
  Divide2/1 -> Add3/1  "AirCtl_qInrLimSmk"
  Add1/1 -> Add2/2  "AirCtl_qSmkHysVal_mp"
  Add/1 -> Add1/2  "AirCtl_qSmkHysCorVal_mp"
  AirCtl_qSmkHys_MAP/1 -> Add1/1  "AirCtl_qSmkHys_mp"
  Divide1/1 -> Add/2  "AirCtl_qEnvPresSmkHysCorVal_mp"
  Divide3/1 -> Add/1  "AirCtl_qEngTempSmkHysCorVal_mp"
  AirCtl_facEngTempSmkHysCor_CUR/1 -> Divide3/2  "AirCtl_facEngTempSmkHysCor_mp"
  AirCtl_qEngTempSmkHysCor_MAP/1 -> Divide3/1  "AirCtl_qEngTempSmkHysCor_mp"
  AirCtl_tEngMon_mp/1 -> AirCtl_facEngTempSmkHysCor_CUR/1
  AirCtl_qEnvPresSmkHysCor_MAP/1 -> Divide1/1  "AirCtl_qEnvPresSmkHysCor_mp"
  InjCtl_qSetUnBal/1 -> AirCtl_qSmkHys_MAP/1, AirCtl_qEngTempSmkHysCor_MAP/1, AirCtl_qEnvPresSmkHysCor_MAP/1, Add3/2
  Epm_nEng/1 -> AirCtl_qSmkHys_MAP/2, AirCtl_qEngTempSmkHysCor_MAP/2, AirCtl_qEnvPresSmkHysCor_MAP/2
  AirCtl_facEnvPresSmkHysCor_CUR/1 -> Divide1/2  "AirCtl_facEnvPresSmkHysCor_mp"
  EnvP_p/1 -> AirCtl_facEnvPresSmkHysCor_CUR/1
  Bit Clear5/1 -> Switch6/3
  Bit Set5/1 -> Switch6/1
  Constant4/1 -> TurnOffDelay2/2
  Logical Operator5/1 -> TurnOnDelay/1  "AirCtl_stDynSwtSmk_mp"
  Relational Operator3/1 -> Logical Operator5/3
  Relational Operator2/1 -> Logical Operator5/1
  Relational Operator1/1 -> Logical Operator5/2
  Constant3/1 -> Relational Operator2/2
  APP_drUnFlt/1 -> Relational Operator2/1
  Constant1/1 -> Relational Operator1/2
  Epm_dnEng/1 -> Relational Operator1/1
  Constant2/1 -> Relational Operator3/2
  InjCtl_dqLead/1 -> Relational Operator3/1
  TurnOnDelay/1 -> TurnOffDelay2/1
  Constant11/1 -> TurnOnDelay/3
  Constant10/1 -> TurnOnDelay/2
  TurnOffDelay2/1 -> Switch6/2

== system AirCtl_Mon/VarDflValCalc_inl9 ==
  note: %1~21对应_CA[1]~_CA[21]
      | 不同关断情况对应选择不同的默认值%
  stMon : Inport
  Constant1 : Constant  Value=AirCtl_rTVADflVal_CA
  Constant6 : Constant  Value=AirCtl_rEGRDflVal_CA
  Selector : Selector  IndexMode=Zero-based  InputPortWidth=30  IndexOptions=Index vector (port)  Indices=[1 3]  OutputSizes=1
  Selector1 : Selector  IndexMode=Zero-based  InputPortWidth=30  IndexOptions=Index vector (port)  Indices=[1 3]  OutputSizes=1
  rEGRDflVal : Outport
  rTVADflVal : Outport  Port=2
  wires:
  Selector/1 -> rEGRDflVal/1
  Selector1/1 -> rTVADflVal/1
  Constant1/1 -> Selector1/1
  Constant6/1 -> Selector/1
  stMon/1 -> Selector/2, Selector1/2

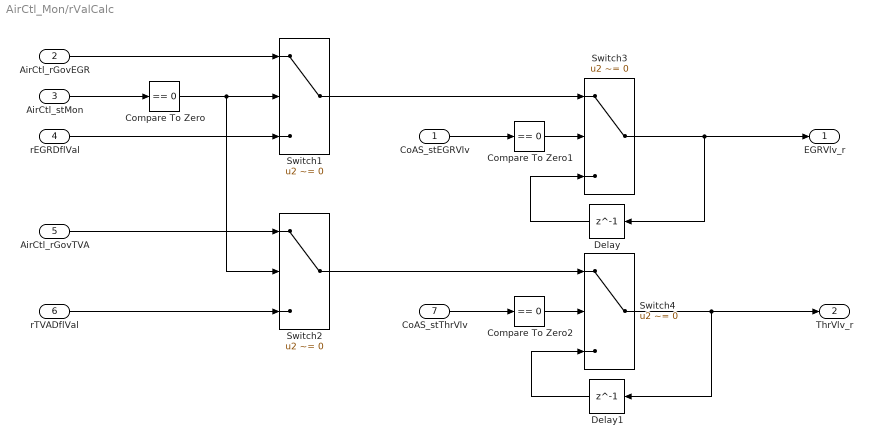
== system AirCtl_Mon/rValCalc ==
  CoAS_stEGRVlv : Inport
  AirCtl_rGovEGR : Inport  Port=2
  AirCtl_stMon : Inport  Port=3
  rEGRDflVal : Inport  Port=4
  AirCtl_rGovTVA : Inport  Port=5
  rTVADflVal : Inport  Port=6
  CoAS_stThrVlv : Inport  Port=7
  Compare To Zero : simulink/Logic and Bit Operations/Compare To Zero  relop===  OutDataTypeStr=boolean
  Compare To Zero1 : simulink/Logic and Bit Operations/Compare To Zero  relop===  OutDataTypeStr=boolean
  Compare To Zero2 : simulink/Logic and Bit Operations/Compare To Zero  relop===  OutDataTypeStr=boolean
  Delay : Delay  DelayLength=1  InitialCondition=0
  Delay1 : Delay  DelayLength=1  InitialCondition=0
  Switch{1..4} (4 alike) : Switch  Criteria=u2 ~= 0  SaturateOnIntegerOverflow=on  InputSameDT=on
  EGRVlv_r : Outport
  ThrVlv_r : Outport  Port=2
  wires:
  CoAS_stEGRVlv/1 -> Compare To Zero1/1
  Delay1/1 -> Switch4/3
  Compare To Zero2/1 -> Switch4/2
  Delay/1 -> Switch3/3
  CoAS_stThrVlv/1 -> Compare To Zero2/1
  rTVADflVal/1 -> Switch2/3
  Switch3/1 -> EGRVlv_r/1, Delay/1
  Compare To Zero1/1 -> Switch3/2
  AirCtl_rGovEGR/1 -> Switch1/1
  rEGRDflVal/1 -> Switch1/3
  Switch2/1 -> Switch4/1
  Compare To Zero/1 -> Switch1/2, Switch2/2
  Switch1/1 -> Switch3/1
  AirCtl_rGovTVA/1 -> Switch2/1
  AirCtl_stMon/1 -> Compare To Zero/1
  Switch4/1 -> Delay1/1, ThrVlv_r/1

== system AirCtl_Mon/CheckPrio/GetBit1 ==
  u : Inport  OutDataTypeStr=uint32
  bit : Inport  Port=2
  GetBit : Stateflow chart  TreatAsAtomicUnit=on
  dataLength : Constant  Value=dataLength  OutDataTypeStr=uint8
  y : Outport  OutDataTypeStr=boolean
  wires:
  dataLength/1 -> GetBit/3(data_length)
  GetBit/1(BitValue) -> y/1
  u/1 -> GetBit/1(Value)
  bit/1 -> GetBit/2(BitPos)

== system AirCtl_Mon/CheckPrio/GetBit10 ==
  u : Inport  OutDataTypeStr=uint32
  bit : Inport  Port=2
  GetBit : Stateflow chart  TreatAsAtomicUnit=on
  dataLength : Constant  Value=dataLength  OutDataTypeStr=uint8
  y : Outport  OutDataTypeStr=boolean
  wires:
  dataLength/1 -> GetBit/3(data_length)
  GetBit/1(BitValue) -> y/1
  u/1 -> GetBit/1(Value)
  bit/1 -> GetBit/2(BitPos)

== system AirCtl_Mon/CheckPrio/GetBit11 ==
  u : Inport  OutDataTypeStr=uint32
  bit : Inport  Port=2
  GetBit : Stateflow chart  TreatAsAtomicUnit=on
  dataLength : Constant  Value=dataLength  OutDataTypeStr=uint8
  y : Outport  OutDataTypeStr=boolean
  wires:
  dataLength/1 -> GetBit/3(data_length)
  GetBit/1(BitValue) -> y/1
  u/1 -> GetBit/1(Value)
  bit/1 -> GetBit/2(BitPos)

== system AirCtl_Mon/CheckPrio/GetBit12 ==
  u : Inport  OutDataTypeStr=uint32
  bit : Inport  Port=2
  GetBit : Stateflow chart  TreatAsAtomicUnit=on
  dataLength : Constant  Value=dataLength  OutDataTypeStr=uint8
  y : Outport  OutDataTypeStr=boolean
  wires:
  dataLength/1 -> GetBit/3(data_length)
  GetBit/1(BitValue) -> y/1
  u/1 -> GetBit/1(Value)
  bit/1 -> GetBit/2(BitPos)

== system AirCtl_Mon/CheckPrio/GetBit13 ==
  u : Inport  OutDataTypeStr=uint32
  bit : Inport  Port=2
  GetBit : Stateflow chart  TreatAsAtomicUnit=on
  dataLength : Constant  Value=dataLength  OutDataTypeStr=uint8
  y : Outport  OutDataTypeStr=boolean
  wires:
  dataLength/1 -> GetBit/3(data_length)
  GetBit/1(BitValue) -> y/1
  u/1 -> GetBit/1(Value)
  bit/1 -> GetBit/2(BitPos)

== system AirCtl_Mon/CheckPrio/GetBit14 ==
  u : Inport  OutDataTypeStr=uint32
  bit : Inport  Port=2
  GetBit : Stateflow chart  TreatAsAtomicUnit=on
  dataLength : Constant  Value=dataLength  OutDataTypeStr=uint8
  y : Outport  OutDataTypeStr=boolean
  wires:
  dataLength/1 -> GetBit/3(data_length)
  GetBit/1(BitValue) -> y/1
  u/1 -> GetBit/1(Value)
  bit/1 -> GetBit/2(BitPos)

== system AirCtl_Mon/CheckPrio/GetBit15 ==
  u : Inport  OutDataTypeStr=uint32
  bit : Inport  Port=2
  GetBit : Stateflow chart  TreatAsAtomicUnit=on
  dataLength : Constant  Value=dataLength  OutDataTypeStr=uint8
  y : Outport  OutDataTypeStr=boolean
  wires:
  dataLength/1 -> GetBit/3(data_length)
  GetBit/1(BitValue) -> y/1
  u/1 -> GetBit/1(Value)
  bit/1 -> GetBit/2(BitPos)

== system AirCtl_Mon/CheckPrio/GetBit16 ==
  u : Inport  OutDataTypeStr=uint32
  bit : Inport  Port=2
  GetBit : Stateflow chart  TreatAsAtomicUnit=on
  dataLength : Constant  Value=dataLength  OutDataTypeStr=uint8
  y : Outport  OutDataTypeStr=boolean
  wires:
  dataLength/1 -> GetBit/3(data_length)
  GetBit/1(BitValue) -> y/1
  u/1 -> GetBit/1(Value)
  bit/1 -> GetBit/2(BitPos)

== system AirCtl_Mon/CheckPrio/GetBit17 ==
  u : Inport  OutDataTypeStr=uint32
  bit : Inport  Port=2
  GetBit : Stateflow chart  TreatAsAtomicUnit=on
  dataLength : Constant  Value=dataLength  OutDataTypeStr=uint8
  y : Outport  OutDataTypeStr=boolean
  wires:
  dataLength/1 -> GetBit/3(data_length)
  GetBit/1(BitValue) -> y/1
  u/1 -> GetBit/1(Value)
  bit/1 -> GetBit/2(BitPos)

== system AirCtl_Mon/CheckPrio/GetBit18 ==
  u : Inport  OutDataTypeStr=uint32
  bit : Inport  Port=2
  GetBit : Stateflow chart  TreatAsAtomicUnit=on
  dataLength : Constant  Value=dataLength  OutDataTypeStr=uint8
  y : Outport  OutDataTypeStr=boolean
  wires:
  dataLength/1 -> GetBit/3(data_length)
  GetBit/1(BitValue) -> y/1
  u/1 -> GetBit/1(Value)
  bit/1 -> GetBit/2(BitPos)

== system AirCtl_Mon/CheckPrio/GetBit19 ==
  u : Inport  OutDataTypeStr=uint32
  bit : Inport  Port=2
  GetBit : Stateflow chart  TreatAsAtomicUnit=on
  dataLength : Constant  Value=dataLength  OutDataTypeStr=uint8
  y : Outport  OutDataTypeStr=boolean
  wires:
  dataLength/1 -> GetBit/3(data_length)
  GetBit/1(BitValue) -> y/1
  u/1 -> GetBit/1(Value)
  bit/1 -> GetBit/2(BitPos)

== system AirCtl_Mon/CheckPrio/GetBit2 ==
  u : Inport  OutDataTypeStr=uint32
  bit : Inport  Port=2
  GetBit : Stateflow chart  TreatAsAtomicUnit=on
  dataLength : Constant  Value=dataLength  OutDataTypeStr=uint8
  y : Outport  OutDataTypeStr=boolean
  wires:
  dataLength/1 -> GetBit/3(data_length)
  GetBit/1(BitValue) -> y/1
  u/1 -> GetBit/1(Value)
  bit/1 -> GetBit/2(BitPos)

== system AirCtl_Mon/CheckPrio/GetBit20 ==
  u : Inport  OutDataTypeStr=uint32
  bit : Inport  Port=2
  GetBit : Stateflow chart  TreatAsAtomicUnit=on
  dataLength : Constant  Value=dataLength  OutDataTypeStr=uint8
  y : Outport  OutDataTypeStr=boolean
  wires:
  dataLength/1 -> GetBit/3(data_length)
  GetBit/1(BitValue) -> y/1
  u/1 -> GetBit/1(Value)
  bit/1 -> GetBit/2(BitPos)

== system AirCtl_Mon/CheckPrio/GetBit21 ==
  u : Inport  OutDataTypeStr=uint32
  bit : Inport  Port=2
  GetBit : Stateflow chart  TreatAsAtomicUnit=on
  dataLength : Constant  Value=dataLength  OutDataTypeStr=uint8
  y : Outport  OutDataTypeStr=boolean
  wires:
  dataLength/1 -> GetBit/3(data_length)
  GetBit/1(BitValue) -> y/1
  u/1 -> GetBit/1(Value)
  bit/1 -> GetBit/2(BitPos)

== system AirCtl_Mon/CheckPrio/GetBit22 ==
  u : Inport  OutDataTypeStr=uint32
  bit : Inport  Port=2
  GetBit : Stateflow chart  TreatAsAtomicUnit=on
  dataLength : Constant  Value=dataLength  OutDataTypeStr=uint8
  y : Outport  OutDataTypeStr=boolean
  wires:
  dataLength/1 -> GetBit/3(data_length)
  GetBit/1(BitValue) -> y/1
  u/1 -> GetBit/1(Value)
  bit/1 -> GetBit/2(BitPos)

== system AirCtl_Mon/CheckPrio/GetBit23 ==
  u : Inport  OutDataTypeStr=uint32
  bit : Inport  Port=2
  GetBit : Stateflow chart  TreatAsAtomicUnit=on
  dataLength : Constant  Value=dataLength  OutDataTypeStr=uint8
  y : Outport  OutDataTypeStr=boolean
  wires:
  dataLength/1 -> GetBit/3(data_length)
  GetBit/1(BitValue) -> y/1
  u/1 -> GetBit/1(Value)
  bit/1 -> GetBit/2(BitPos)

== system AirCtl_Mon/CheckPrio/GetBit24 ==
  u : Inport  OutDataTypeStr=uint32
  bit : Inport  Port=2
  GetBit : Stateflow chart  TreatAsAtomicUnit=on
  dataLength : Constant  Value=dataLength  OutDataTypeStr=uint8
  y : Outport  OutDataTypeStr=boolean
  wires:
  dataLength/1 -> GetBit/3(data_length)
  GetBit/1(BitValue) -> y/1
  u/1 -> GetBit/1(Value)
  bit/1 -> GetBit/2(BitPos)

== system AirCtl_Mon/CheckPrio/GetBit25 ==
  u : Inport  OutDataTypeStr=uint32
  bit : Inport  Port=2
  GetBit : Stateflow chart  TreatAsAtomicUnit=on
  dataLength : Constant  Value=dataLength  OutDataTypeStr=uint8
  y : Outport  OutDataTypeStr=boolean
  wires:
  dataLength/1 -> GetBit/3(data_length)
  GetBit/1(BitValue) -> y/1
  u/1 -> GetBit/1(Value)
  bit/1 -> GetBit/2(BitPos)

== system AirCtl_Mon/CheckPrio/GetBit26 ==
  u : Inport  OutDataTypeStr=uint32
  bit : Inport  Port=2
  GetBit : Stateflow chart  TreatAsAtomicUnit=on
  dataLength : Constant  Value=dataLength  OutDataTypeStr=uint8
  y : Outport  OutDataTypeStr=boolean
  wires:
  dataLength/1 -> GetBit/3(data_length)
  GetBit/1(BitValue) -> y/1
  u/1 -> GetBit/1(Value)
  bit/1 -> GetBit/2(BitPos)

== system AirCtl_Mon/CheckPrio/GetBit29 ==
  u : Inport  OutDataTypeStr=uint32
  bit : Inport  Port=2
  GetBit : Stateflow chart  TreatAsAtomicUnit=on
  dataLength : Constant  Value=dataLength  OutDataTypeStr=uint8
  y : Outport  OutDataTypeStr=boolean
  wires:
  dataLength/1 -> GetBit/3(data_length)
  GetBit/1(BitValue) -> y/1
  u/1 -> GetBit/1(Value)
  bit/1 -> GetBit/2(BitPos)

== system AirCtl_Mon/CheckPrio/GetBit3 ==
  u : Inport  OutDataTypeStr=uint32
  bit : Inport  Port=2
  GetBit : Stateflow chart  TreatAsAtomicUnit=on
  dataLength : Constant  Value=dataLength  OutDataTypeStr=uint8
  y : Outport  OutDataTypeStr=boolean
  wires:
  dataLength/1 -> GetBit/3(data_length)
  GetBit/1(BitValue) -> y/1
  u/1 -> GetBit/1(Value)
  bit/1 -> GetBit/2(BitPos)

== system AirCtl_Mon/CheckPrio/GetBit4 ==
  u : Inport  OutDataTypeStr=uint32
  bit : Inport  Port=2
  GetBit : Stateflow chart  TreatAsAtomicUnit=on
  dataLength : Constant  Value=dataLength  OutDataTypeStr=uint8
  y : Outport  OutDataTypeStr=boolean
  wires:
  dataLength/1 -> GetBit/3(data_length)
  GetBit/1(BitValue) -> y/1
  u/1 -> GetBit/1(Value)
  bit/1 -> GetBit/2(BitPos)

== system AirCtl_Mon/CheckPrio/GetBit5 ==
  u : Inport  OutDataTypeStr=uint32
  bit : Inport  Port=2
  GetBit : Stateflow chart  TreatAsAtomicUnit=on
  dataLength : Constant  Value=dataLength  OutDataTypeStr=uint8
  y : Outport  OutDataTypeStr=boolean
  wires:
  dataLength/1 -> GetBit/3(data_length)
  GetBit/1(BitValue) -> y/1
  u/1 -> GetBit/1(Value)
  bit/1 -> GetBit/2(BitPos)

== system AirCtl_Mon/CheckPrio/GetBit6 ==
  u : Inport  OutDataTypeStr=uint32
  bit : Inport  Port=2
  GetBit : Stateflow chart  TreatAsAtomicUnit=on
  dataLength : Constant  Value=dataLength  OutDataTypeStr=uint8
  y : Outport  OutDataTypeStr=boolean
  wires:
  dataLength/1 -> GetBit/3(data_length)
  GetBit/1(BitValue) -> y/1
  u/1 -> GetBit/1(Value)
  bit/1 -> GetBit/2(BitPos)

== system AirCtl_Mon/CheckPrio/GetBit7 ==
  u : Inport  OutDataTypeStr=uint32
  bit : Inport  Port=2
  GetBit : Stateflow chart  TreatAsAtomicUnit=on
  dataLength : Constant  Value=dataLength  OutDataTypeStr=uint8
  y : Outport  OutDataTypeStr=boolean
  wires:
  dataLength/1 -> GetBit/3(data_length)
  GetBit/1(BitValue) -> y/1
  u/1 -> GetBit/1(Value)
  bit/1 -> GetBit/2(BitPos)

== system AirCtl_Mon/CheckPrio/GetBit8 ==
  u : Inport  OutDataTypeStr=uint32
  bit : Inport  Port=2
  GetBit : Stateflow chart  TreatAsAtomicUnit=on
  dataLength : Constant  Value=dataLength  OutDataTypeStr=uint8
  y : Outport  OutDataTypeStr=boolean
  wires:
  dataLength/1 -> GetBit/3(data_length)
  GetBit/1(BitValue) -> y/1
  u/1 -> GetBit/1(Value)
  bit/1 -> GetBit/2(BitPos)

== system AirCtl_Mon/CheckPrio/GetBit9 ==
  u : Inport  OutDataTypeStr=uint32
  bit : Inport  Port=2
  GetBit : Stateflow chart  TreatAsAtomicUnit=on
  dataLength : Constant  Value=dataLength  OutDataTypeStr=uint8
  y : Outport  OutDataTypeStr=boolean
  wires:
  dataLength/1 -> GetBit/3(data_length)
  GetBit/1(BitValue) -> y/1
  u/1 -> GetBit/1(Value)
  bit/1 -> GetBit/2(BitPos)

== system AirCtl_Mon/CheckPrio/If Action Subsystem ==
  note: %[1]~[21]%
  Action Port : ActionPort  InitializeStates=reset  ActionType=then
  Constant1 : Constant  OutDataTypeStr=uint8
  Constant6 : Constant  Value=AirCtl_stPrioMon_CA
  Selector2 : Selector  IndexMode=Zero-based  InputPortWidth=30  IndexOptions=Index vector (port)  Indices=[1 3]  OutputSizes=1
  priority1 : Outport  OutputWhenDisabled=reset  InitialOutput=0
  wires:
  Selector2/1 -> priority1/1
  Constant1/1 -> Selector2/2
  Constant6/1 -> Selector2/1

== system AirCtl_Mon/CheckPrio/If Action Subsystem1 ==
  note: %[1]~[21]%
  Action Port : ActionPort  InitializeStates=reset  ActionType=then
  Constant1 : Constant  Value=2  OutDataTypeStr=uint8
  Constant6 : Constant  Value=AirCtl_stPrioMon_CA
  Selector2 : Selector  IndexMode=Zero-based  InputPortWidth=30  IndexOptions=Index vector (port)  Indices=[1 3]  OutputSizes=1
  priority2 : Outport  OutputWhenDisabled=reset  InitialOutput=0
  wires:
  Constant6/1 -> Selector2/1
  Constant1/1 -> Selector2/2
  Selector2/1 -> priority2/1

== system AirCtl_Mon/CheckPrio/If Action Subsystem10 ==
  note: %[1]~[21]%
  Action Port : ActionPort  InitializeStates=reset  ActionType=then
  Constant1 : Constant  Value=11  OutDataTypeStr=uint8
  Constant6 : Constant  Value=AirCtl_stPrioMon_CA
  Selector2 : Selector  IndexMode=Zero-based  InputPortWidth=30  IndexOptions=Index vector (port)  Indices=[1 3]  OutputSizes=1
  priority11 : Outport  OutputWhenDisabled=reset  InitialOutput=0
  wires:
  Constant6/1 -> Selector2/1
  Constant1/1 -> Selector2/2
  Selector2/1 -> priority11/1

== system AirCtl_Mon/CheckPrio/If Action Subsystem11 ==
  note: %[1]~[21]%
  Action Port : ActionPort  InitializeStates=reset  ActionType=then
  Constant1 : Constant  Value=12  OutDataTypeStr=uint8
  Constant6 : Constant  Value=AirCtl_stPrioMon_CA
  Selector2 : Selector  IndexMode=Zero-based  InputPortWidth=30  IndexOptions=Index vector (port)  Indices=[1 3]  OutputSizes=1
  priority12 : Outport  OutputWhenDisabled=reset  InitialOutput=0
  wires:
  Selector2/1 -> priority12/1
  Constant1/1 -> Selector2/2
  Constant6/1 -> Selector2/1

== system AirCtl_Mon/CheckPrio/If Action Subsystem12 ==
  note: %[1]~[21]%
  Action Port : ActionPort  InitializeStates=reset  ActionType=then
  Constant1 : Constant  Value=13  OutDataTypeStr=uint8
  Constant6 : Constant  Value=AirCtl_stPrioMon_CA
  Selector2 : Selector  IndexMode=Zero-based  InputPortWidth=30  IndexOptions=Index vector (port)  Indices=[1 3]  OutputSizes=1
  priority13 : Outport  OutputWhenDisabled=reset  InitialOutput=0
  wires:
  Constant6/1 -> Selector2/1
  Constant1/1 -> Selector2/2
  Selector2/1 -> priority13/1

== system AirCtl_Mon/CheckPrio/If Action Subsystem13 ==
  note: %[1]~[21]%
  Action Port : ActionPort  InitializeStates=reset  ActionType=then
  Constant1 : Constant  Value=14  OutDataTypeStr=uint8
  Constant6 : Constant  Value=AirCtl_stPrioMon_CA
  Selector2 : Selector  IndexMode=Zero-based  InputPortWidth=30  IndexOptions=Index vector (port)  Indices=[1 3]  OutputSizes=1
  priority14 : Outport  OutputWhenDisabled=reset  InitialOutput=0
  wires:
  Selector2/1 -> priority14/1
  Constant1/1 -> Selector2/2
  Constant6/1 -> Selector2/1

== system AirCtl_Mon/CheckPrio/If Action Subsystem14 ==
  note: %[1]~[21]%
  Action Port : ActionPort  InitializeStates=reset  ActionType=then
  Constant1 : Constant  Value=15  OutDataTypeStr=uint8
  Constant6 : Constant  Value=AirCtl_stPrioMon_CA
  Selector2 : Selector  IndexMode=Zero-based  InputPortWidth=30  IndexOptions=Index vector (port)  Indices=[1 3]  OutputSizes=1
  priority15 : Outport  OutputWhenDisabled=reset  InitialOutput=0
  wires:
  Constant6/1 -> Selector2/1
  Constant1/1 -> Selector2/2
  Selector2/1 -> priority15/1

== system AirCtl_Mon/CheckPrio/If Action Subsystem15 ==
  note: %[1]~[21]%
  Action Port : ActionPort  InitializeStates=reset  ActionType=then
  Constant1 : Constant  Value=16  OutDataTypeStr=uint8
  Constant6 : Constant  Value=AirCtl_stPrioMon_CA
  Selector2 : Selector  IndexMode=Zero-based  InputPortWidth=30  IndexOptions=Index vector (port)  Indices=[1 3]  OutputSizes=1
  priority16 : Outport  OutputWhenDisabled=reset  InitialOutput=0
  wires:
  Selector2/1 -> priority16/1
  Constant1/1 -> Selector2/2
  Constant6/1 -> Selector2/1

== system AirCtl_Mon/CheckPrio/If Action Subsystem16 ==
  note: %[1]~[21]%
  Action Port : ActionPort  InitializeStates=reset  ActionType=then
  Constant1 : Constant  Value=17  OutDataTypeStr=uint8
  Constant6 : Constant  Value=AirCtl_stPrioMon_CA
  Selector2 : Selector  IndexMode=Zero-based  InputPortWidth=30  IndexOptions=Index vector (port)  Indices=[1 3]  OutputSizes=1
  priority17 : Outport  OutputWhenDisabled=reset  InitialOutput=0
  wires:
  Constant6/1 -> Selector2/1
  Constant1/1 -> Selector2/2
  Selector2/1 -> priority17/1

== system AirCtl_Mon/CheckPrio/If Action Subsystem17 ==
  note: %[1]~[21]%
  Action Port : ActionPort  InitializeStates=reset  ActionType=then
  Constant1 : Constant  Value=18  OutDataTypeStr=uint8
  Constant6 : Constant  Value=AirCtl_stPrioMon_CA
  Selector2 : Selector  IndexMode=Zero-based  InputPortWidth=30  IndexOptions=Index vector (port)  Indices=[1 3]  OutputSizes=1
  priority18 : Outport  OutputWhenDisabled=reset  InitialOutput=0
  wires:
  Selector2/1 -> priority18/1
  Constant1/1 -> Selector2/2
  Constant6/1 -> Selector2/1

== system AirCtl_Mon/CheckPrio/If Action Subsystem18 ==
  note: %[1]~[21]%
  Action Port : ActionPort  InitializeStates=reset  ActionType=then
  Constant1 : Constant  Value=20  OutDataTypeStr=uint8
  Constant6 : Constant  Value=AirCtl_stPrioMon_CA
  Selector2 : Selector  IndexMode=Zero-based  InputPortWidth=30  IndexOptions=Index vector (port)  Indices=[1 3]  OutputSizes=1
  priority20 : Outport  OutputWhenDisabled=reset  InitialOutput=0
  wires:
  Constant6/1 -> Selector2/1
  Constant1/1 -> Selector2/2
  Selector2/1 -> priority20/1

== system AirCtl_Mon/CheckPrio/If Action Subsystem19 ==
  note: %[1]~[21]%
  Action Port : ActionPort  InitializeStates=reset  ActionType=then
  Constant1 : Constant  Value=21  OutDataTypeStr=uint8
  Constant6 : Constant  Value=AirCtl_stPrioMon_CA
  Selector2 : Selector  IndexMode=Zero-based  InputPortWidth=30  IndexOptions=Index vector (port)  Indices=[1 3]  OutputSizes=1
  priority21 : Outport  OutputWhenDisabled=reset  InitialOutput=0
  wires:
  Selector2/1 -> priority21/1
  Constant1/1 -> Selector2/2
  Constant6/1 -> Selector2/1

== system AirCtl_Mon/CheckPrio/If Action Subsystem2 ==
  note: %[1]~[21]%
  Action Port : ActionPort  InitializeStates=reset  ActionType=then
  Constant1 : Constant  Value=3  OutDataTypeStr=uint8
  Constant6 : Constant  Value=AirCtl_stPrioMon_CA
  Selector2 : Selector  IndexMode=Zero-based  InputPortWidth=30  IndexOptions=Index vector (port)  Indices=[1 3]  OutputSizes=1
  priority3 : Outport  OutputWhenDisabled=reset  InitialOutput=0
  wires:
  Selector2/1 -> priority3/1
  Constant1/1 -> Selector2/2
  Constant6/1 -> Selector2/1
